simulink model "sistema"  (R2022a)
settings: Solver=ode1  StartTime=0.0  StopTime=tfinal  FixedStep=tstep  RelTol=1e-3
undefined symbols (not defined in the file or in its folder): ref_speed, wp_index_lim, wp_lat, wp_long, wp_time
libraries: robotmobilelib x1
settings Model: Creator=rodri  LastModifiedBy=rodri
settings DataIOCC: ExternalInput=[t2, u2]  SaveFormat=StructureWithTime  SignalLogging=off  DSMLogging=off  InspectSignalLogs=on  ReturnWorkspaceOutputs=off

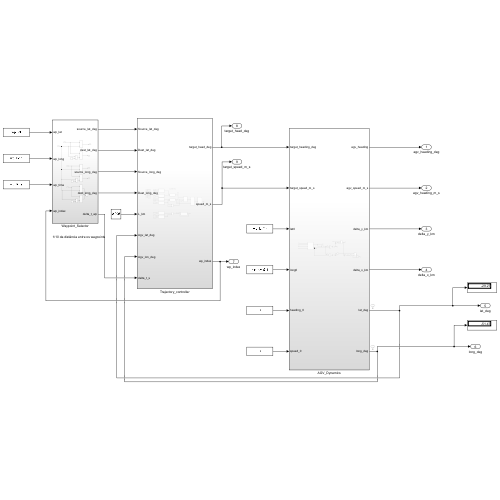
[thumbnail: Simulink's stored preview of the top-level diagram]
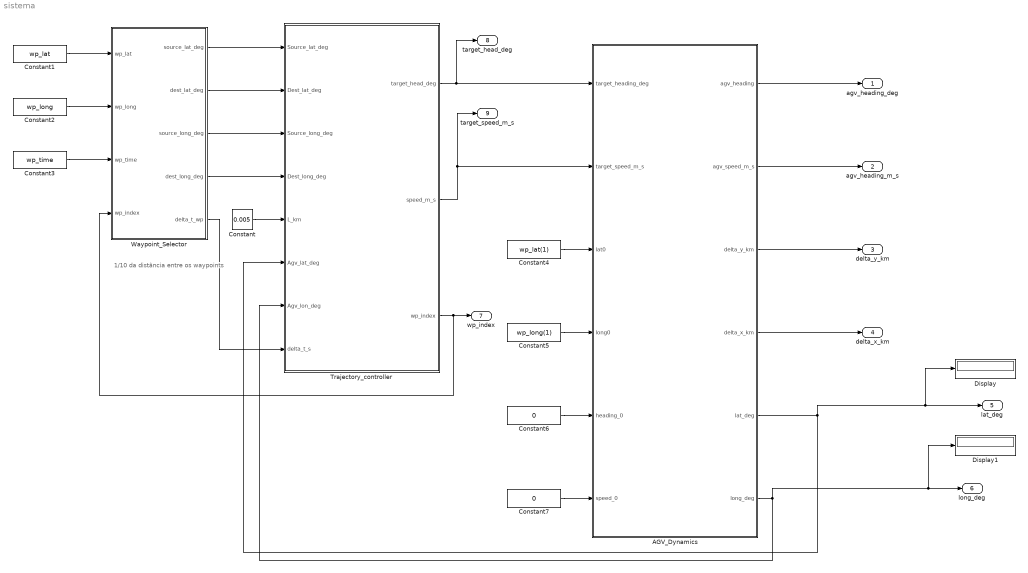
== system sistema ==
  note: 1/10 da distância entre os waypoints
  AGV_Dynamics : Subsystem
  Constant : Constant  Value=0.005
  Constant1 : Constant  Value=wp_lat
  Constant2 : Constant  Value=wp_long
  Constant3 : Constant  Value=wp_time
  Constant4 : Constant  Value=wp_lat(1)
  Constant5 : Constant  Value=wp_long(1)
  Constant6 : Constant  Value=0
  Constant7 : Constant  Value=0
  Display : Display
  Display1 : Display
  Trajectory_controller : Subsystem
  Waypoint_Selector : Subsystem
  agv_heading_deg : Outport
  agv_heading_m_s : Outport  Port=2
  delta_y_km : Outport  Port=3
  delta_x_km : Outport  Port=4
  lat_deg : Outport  Port=5
  long_deg : Outport  Port=6
  wp_index : Outport  Port=7
  target_head_deg : Outport  Port=8
  target_speed_m_s : Outport  Port=9
  wires:
  Waypoint_Selector/1(source_lat_deg) -> Trajectory_controller/1(Source_lat_deg)
  Waypoint_Selector/2(dest_lat_deg) -> Trajectory_controller/2(Dest_lat_deg)
  Waypoint_Selector/3(source_long_deg) -> Trajectory_controller/3(Source_long_deg)
  Waypoint_Selector/4(dest_long_deg) -> Trajectory_controller/4(Dest_long_deg)
  Constant/1 -> Trajectory_controller/5(L_km)
  Constant1/1 -> Waypoint_Selector/1(wp_lat)
  Constant2/1 -> Waypoint_Selector/2(wp_long)
  Constant3/1 -> Waypoint_Selector/3(wp_time)
  Waypoint_Selector/5(delta_t_wp) -> Trajectory_controller/8(delta_t_s)
  Trajectory_controller/3(wp_index) -> Waypoint_Selector/4(wp_index), wp_index/1
  Trajectory_controller/1(target_head_deg) -> target_head_deg/1, AGV_Dynamics/1(target_heading_deg)
  Trajectory_controller/2(speed_m_s) -> target_speed_m_s/1, AGV_Dynamics/2(target_speed_m_s)
  AGV_Dynamics/5(lat_deg) -> Display/1, lat_deg/1, Trajectory_controller/6(Agv_lat_deg)
  AGV_Dynamics/6(long_deg) -> Display1/1, long_deg/1, Trajectory_controller/7(Agv_lon_deg)
  AGV_Dynamics/1(agv_heading) -> agv_heading_deg/1
  AGV_Dynamics/2(agv_speed_m_s) -> agv_heading_m_s/1
  AGV_Dynamics/3(delta_y_km) -> delta_y_km/1
  AGV_Dynamics/4(delta_x_km) -> delta_x_km/1
  Constant4/1 -> AGV_Dynamics/3(lat0)
  Constant5/1 -> AGV_Dynamics/4(long0)
  Constant6/1 -> AGV_Dynamics/5(heading_0)
  Constant7/1 -> AGV_Dynamics/6(speed_0)

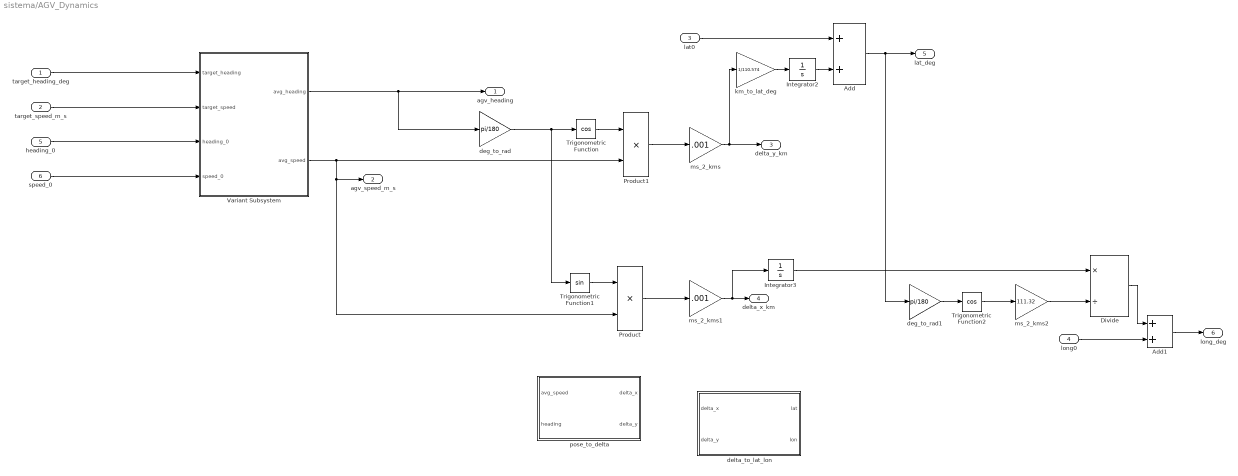
== system sistema/AGV_Dynamics ==
  target_heading_deg : Inport
  target_speed_m_s : Inport  Port=2
  lat0 : Inport  Port=3
  long0 : Inport  Port=4
  heading_0 : Inport  Port=5
  speed_0 : Inport  Port=6
  Add : Sum
  Add1 : Sum
  Divide : Product  Inputs=*/
  Integrator2 : Integrator
  Integrator3 : Integrator
  Product : Product
  Product1 : Product
  Trigonometric Function : Trigonometry  Operator=cos
  Trigonometric Function1 : Trigonometry
  Trigonometric Function2 : Trigonometry  Operator=cos
  Variant Subsystem : Subsystem  Variant=on
  deg_to_rad : Gain  Gain=pi/180
  deg_to_rad1 : Gain  Gain=pi/180
  delta_to_lat_lon : MATLAB Function  TreatAsAtomicUnit=on
  km_to_lat_deg : Gain  Gain=1/110.574
  ms_2_kms : Gain  Gain=.001
  ms_2_kms1 : Gain  Gain=.001
  ms_2_kms2 : Gain  Gain=111.32
  pose_to_delta : MATLAB Function  TreatAsAtomicUnit=on
  agv_heading : Outport
  agv_speed_m_s : Outport  Port=2
  delta_y_km : Outport  Port=3
  delta_x_km : Outport  Port=4
  lat_deg : Outport  Port=5
  long_deg : Outport  Port=6
  wires:
  deg_to_rad/1 -> Trigonometric Function1/1, Trigonometric Function/1
  Trigonometric Function1/1 -> Product/1
  Product/1 -> ms_2_kms1/1
  Trigonometric Function/1 -> Product1/1
  Product1/1 -> ms_2_kms/1
  ms_2_kms/1 -> delta_y_km/1, km_to_lat_deg/1
  ms_2_kms1/1 -> Integrator3/1, delta_x_km/1
  lat0/1 -> Add/1
  km_to_lat_deg/1 -> Integrator2/1
  Add/1 -> deg_to_rad1/1, lat_deg/1
  deg_to_rad1/1 -> Trigonometric Function2/1
  Trigonometric Function2/1 -> ms_2_kms2/1
  long0/1 -> Add1/2
  Divide/1 -> Add1/1
  ms_2_kms2/1 -> Divide/2
  Add1/1 -> long_deg/1
  Integrator3/1 -> Divide/1
  Integrator2/1 -> Add/2
  Variant Subsystem/1(avg_heading) -> deg_to_rad/1, agv_heading/1
  Variant Subsystem/2(avg_speed) -> Product/2, agv_speed_m_s/1, Product1/2
  target_heading_deg/1 -> Variant Subsystem/1(target_heading)
  target_speed_m_s/1 -> Variant Subsystem/2(target_speed)
  heading_0/1 -> Variant Subsystem/3(heading_0)
  speed_0/1 -> Variant Subsystem/4(speed_0)

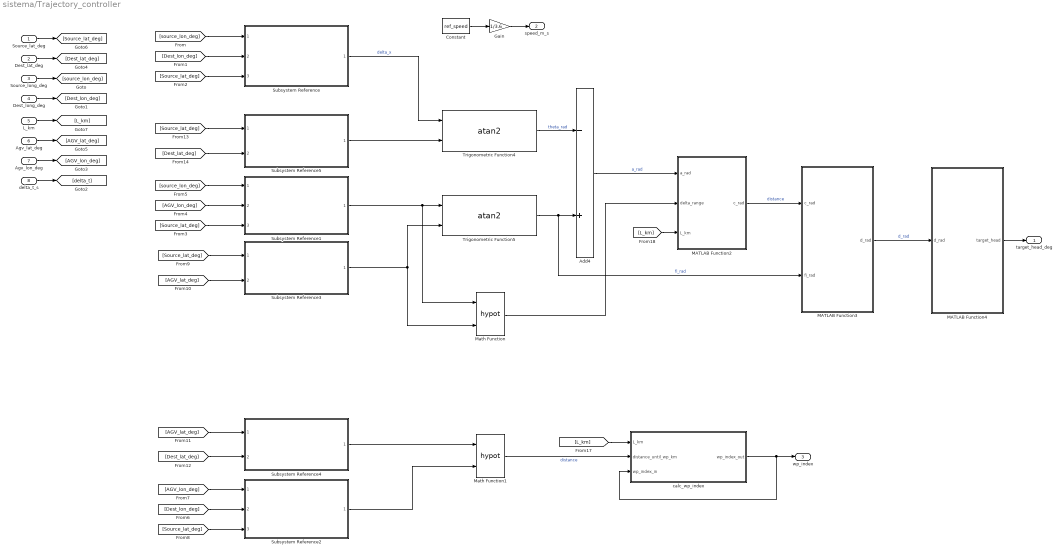
== system sistema/Trajectory_controller ==
  Source_lat_deg : Inport
  Dest_lat_deg : Inport  Port=2
  Source_long_deg : Inport  Port=3
  Dest_long_deg : Inport  Port=4
  L_km : Inport  Port=5
  Agv_lat_deg : Inport  Port=6
  Agv_lon_deg : Inport  Port=7
  delta_t_s : Inport  Port=8
  Add4 : Sum  Inputs=-+
  Constant : Constant  Value=ref_speed
  Gain : Gain  Gain=1/3.6
  MATLAB Function2 : MATLAB Function  TreatAsAtomicUnit=on
  MATLAB Function3 : MATLAB Function  TreatAsAtomicUnit=on
  MATLAB Function4 : MATLAB Function  TreatAsAtomicUnit=on
  Math Function : Math  Operator=hypot
  Math Function1 : Math  Operator=hypot
  Subsystem Reference : Subsystem  ReferencedSubsystem=long_deg_to_km
  Subsystem Reference1 : Subsystem  ReferencedSubsystem=long_deg_to_km
  Subsystem Reference2 : Subsystem  ReferencedSubsystem=long_deg_to_km
  Subsystem Reference3 : Subsystem  ReferencedSubsystem=lat_deg_to_km
  Subsystem Reference4 : Subsystem  ReferencedSubsystem=lat_deg_to_km
  Subsystem Reference5 : Subsystem  ReferencedSubsystem=lat_deg_to_km
  Trigonometric Function4 : Trigonometry  Operator=atan2
  Trigonometric Function5 : Trigonometry  Operator=atan2
  calc_wp_index : Subsystem
  target_head_deg : Outport
  speed_m_s : Outport  Port=2  Unit=m/s
  wp_index : Outport  Port=3
  wires:
  MATLAB Function4/1(target_head) -> target_head_deg/1
  Math Function1/1 -> calc_wp_index/2(distance_until_wp_km)  "distance"
  calc_wp_index/1(wp_index_out) -> calc_wp_index/3(wp_index_in), wp_index/1
  [source_lon_deg] -> Subsystem Reference/1
  [Dest_lon_deg] -> Subsystem Reference/2
  [Source_lat_deg] -> Subsystem Reference/3
  [Source_lat_deg] -> Subsystem Reference1/3
  [AGV_lon_deg] -> Subsystem Reference1/2
  [source_lon_deg] -> Subsystem Reference1/1
  [Dest_lon_deg] -> Subsystem Reference2/2
  [AGV_lon_deg] -> Subsystem Reference2/1
  [Source_lat_deg] -> Subsystem Reference2/3
  [Source_lat_deg] -> Subsystem Reference3/1
  [AGV_lat_deg] -> Subsystem Reference3/2
  [Dest_lat_deg] -> Subsystem Reference4/2
  [AGV_lat_deg] -> Subsystem Reference4/1
  Gain/1 -> speed_m_s/1
  [Source_lat_deg] -> Subsystem Reference5/1
  [Dest_lat_deg] -> Subsystem Reference5/2
  Trigonometric Function4/1 -> Add4/1  "theta_rad"
  Trigonometric Function5/1 -> MATLAB Function3/2(fi_rad), Add4/2  "fi_rad"
  Source_long_deg/1 -> [source_lon_deg]
  Dest_long_deg/1 -> [Dest_lon_deg]
  Source_lat_deg/1 -> [Source_lat_deg]
  Dest_lat_deg/1 -> [Dest_lat_deg]
  Agv_lat_deg/1 -> [AGV_lat_deg]
  Agv_lon_deg/1 -> [AGV_lon_deg]
  delta_t_s/1 -> [delta_t]
  L_km/1 -> [L_km]
  Subsystem Reference/1 -> Trigonometric Function4/1  "delta_x"
  Subsystem Reference5/1 -> Trigonometric Function4/2
  Subsystem Reference1/1 -> Math Function/1, Trigonometric Function5/1
  Subsystem Reference3/1 -> Math Function/2, Trigonometric Function5/2
  Subsystem Reference4/1 -> Math Function1/1
  Subsystem Reference2/1 -> Math Function1/2
  [L_km] -> calc_wp_index/1(L_km)
  Add4/1 -> MATLAB Function2/1(a_rad)  "a_rad"
  MATLAB Function2/1(c_rad) -> MATLAB Function3/1(c_rad)  "distance"
  Math Function/1 -> MATLAB Function2/2(delta_range)
  [L_km] -> MATLAB Function2/3(L_km)
  MATLAB Function3/1(d_rad) -> MATLAB Function4/1(d_rad)  "d_rad"
  Constant/1 -> Gain/1

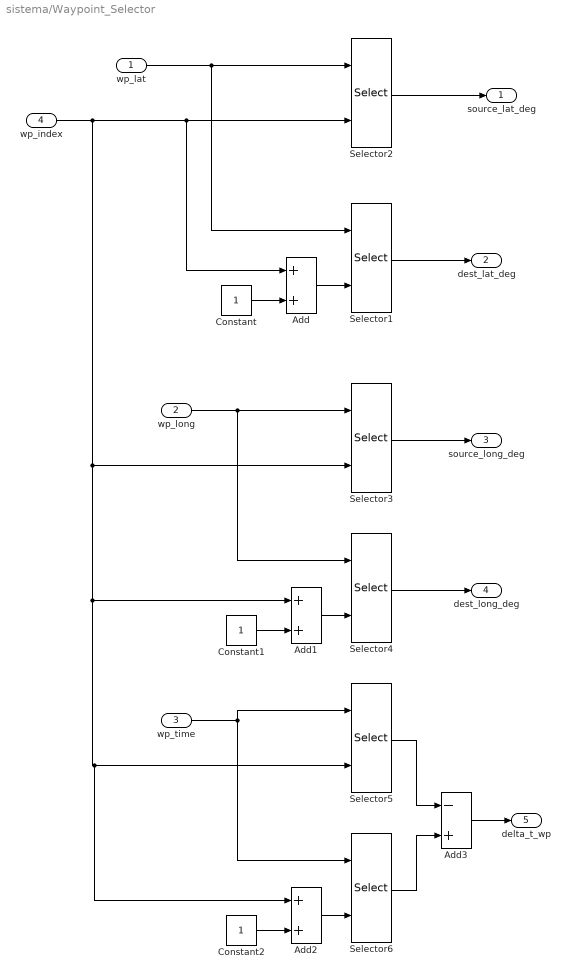
== system sistema/Waypoint_Selector ==
  wp_lat : Inport
  wp_long : Inport  Port=2
  wp_time : Inport  Port=3
  wp_index : Inport  Port=4
  Add : Sum
  Add1 : Sum
  Add2 : Sum
  Add3 : Sum  Inputs=-+
  Constant : Constant
  Constant1 : Constant
  Constant2 : Constant
  Selector{1..6} (6 alike) : Selector  InputPortWidth=num_of_wps  IndexOptions=Index vector (port)  Indices=[1 3]  OutputSizes=1
  source_lat_deg : Outport
  dest_lat_deg : Outport  Port=2
  source_long_deg : Outport  Port=3
  dest_long_deg : Outport  Port=4
  delta_t_wp : Outport  Port=5
  wires:
  Selector2/1 -> source_lat_deg/1
  Selector1/1 -> dest_lat_deg/1
  wp_lat/1 -> Selector2/1, Selector1/1
  Add/1 -> Selector1/2
  Constant/1 -> Add/2
  Selector3/1 -> source_long_deg/1
  Selector4/1 -> dest_long_deg/1
  wp_long/1 -> Selector4/1, Selector3/1
  Constant1/1 -> Add1/2
  Add1/1 -> Selector4/2
  Add2/1 -> Selector6/2
  Constant2/1 -> Add2/2
  wp_time/1 -> Selector5/1, Selector6/1
  wp_index/1 -> Add2/1, Selector5/2, Add1/1, Selector3/2, Selector2/2, Add/1
  Selector5/1 -> Add3/1
  Selector6/1 -> Add3/2
  Add3/1 -> delta_t_wp/1

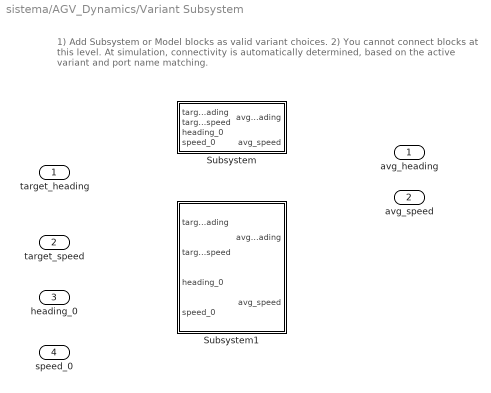
== system sistema/AGV_Dynamics/Variant Subsystem ==
  note: 1) Add Subsystem or Model blocks as valid variant choices.
      | 2) You cannot connect blocks at this level. At simulation, connectivity is automatically
      | determined, based on the active variant and port name matching.
  target_heading : Inport  Unit=deg
  target_speed : Inport  Port=2  Unit=m/s
  heading_0 : Inport  Port=3  Unit=m/s
  speed_0 : Inport  Port=4  Unit=m/s
  Subsystem : Subsystem  VariantControl=DYNMODE == 1
  Subsystem1 : Subsystem  VariantControl=DYNMODE == 2
  avg_heading : Outport
  avg_speed : Outport  Port=2

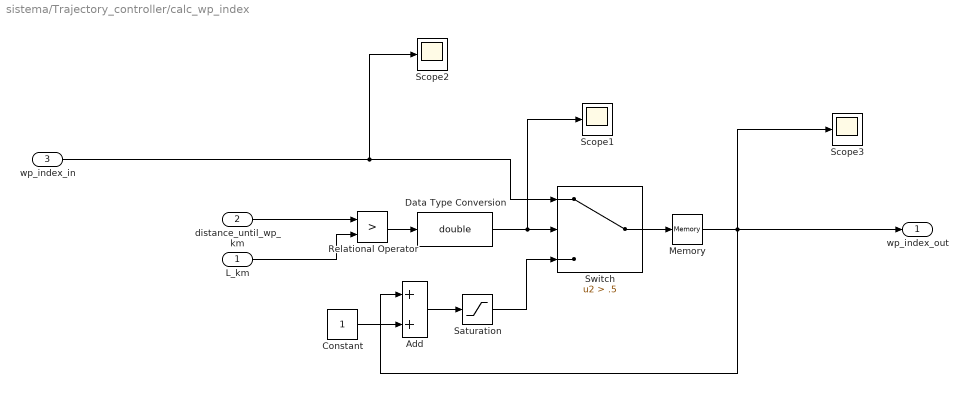
== system sistema/Trajectory_controller/calc_wp_index ==
  L_km : Inport
  distance_until_wp_km : Inport  Port=2
  wp_index_in : Inport  Port=3
  Add : Sum
  Constant : Constant
  Data Type Conversion : DataTypeConversion  OutDataTypeStr=double  SaturateOnIntegerOverflow=off  RndMeth=Floor
  Memory : Memory  InitialCondition=1
  Relational Operator : RelationalOperator  Operator=>  OutDataTypeStr=boolean  RndMeth=Simplest  InputSameDT=off
  Saturation : Saturate  UpperLimit=wp_index_lim  LowerLimit=1
  Scope1 : Scope
  Scope2 : Scope
  Scope3 : Scope
  Switch : Switch  Criteria=u2 > Threshold  Threshold=.5  SaturateOnIntegerOverflow=off  InputSameDT=off
  wp_index_out : Outport
  wires:
  distance_until_wp_km/1 -> Relational Operator/1
  L_km/1 -> Relational Operator/2
  Relational Operator/1 -> Data Type Conversion/1
  Data Type Conversion/1 -> Scope1/1, Switch/2
  Switch/1 -> Memory/1
  Memory/1 -> Add/1, Scope3/1, wp_index_out/1
  wp_index_in/1 -> Scope2/1, Switch/1
  Add/1 -> Saturation/1
  Constant/1 -> Add/2
  Saturation/1 -> Switch/3

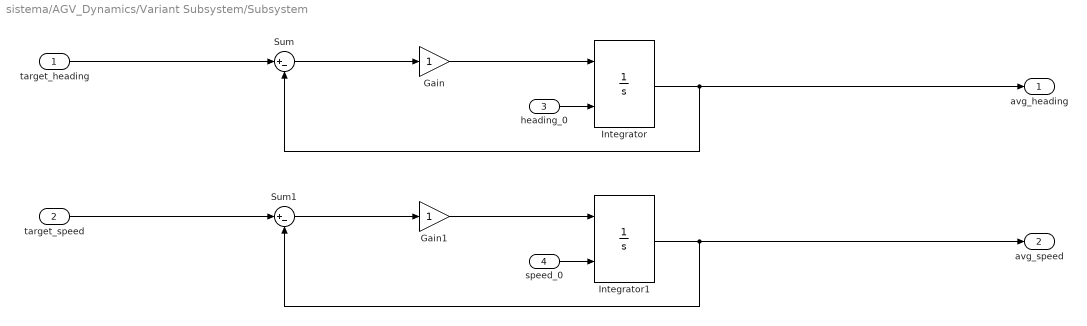
== system sistema/AGV_Dynamics/Variant Subsystem/Subsystem ==
  target_heading : Inport
  target_speed : Inport  Port=2
  heading_0 : Inport  Port=3
  speed_0 : Inport  Port=4
  Gain : Gain
  Gain1 : Gain
  Integrator : Integrator  InitialConditionSource=external
  Integrator1 : Integrator  InitialConditionSource=external
  Sum : Sum  Inputs=|+-
  Sum1 : Sum  Inputs=|+-
  avg_heading : Outport
  avg_speed : Outport  Port=2
  wires:
  target_speed/1 -> Sum1/1
  heading_0/1 -> Integrator/2
  Sum/1 -> Gain/1
  target_heading/1 -> Sum/1
  Integrator1/1 -> Sum1/2, avg_speed/1
  Gain1/1 -> Integrator1/1
  Sum1/1 -> Gain1/1
  Integrator/1 -> avg_heading/1, Sum/2
  Gain/1 -> Integrator/1
  speed_0/1 -> Integrator1/2

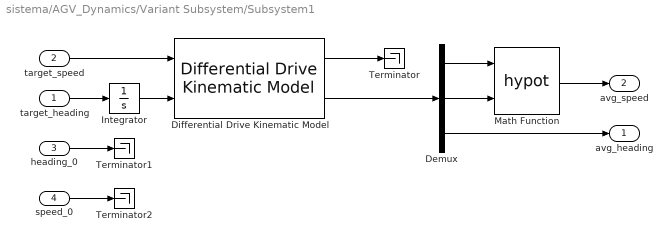
== system sistema/AGV_Dynamics/Variant Subsystem/Subsystem1 ==
  target_heading : Inport
  target_speed : Inport  Port=2
  heading_0 : Inport  Port=3
  speed_0 : Inport  Port=4
  Demux : Demux  Outputs=3
  Differential Drive Kinematic Model : robotmobilelib/Differential Drive Kinematic Model  VehicleInputs=Vehicle Speed & Heading Angular Velocity  WheelRadius=0.05  WheelSpeedRange=[-18, 18]  TrackWidth=0.8  InitialState=[0; 0; 0]  SimulateUsing=Interpreted execution
      settings: SourceProductBaseCode=RO
  Integrator : Integrator
  Math Function : Math  Operator=hypot
  Terminator : Terminator
  Terminator1 : Terminator
  Terminator2 : Terminator
  avg_heading : Outport
  avg_speed : Outport  Port=2
  wires:
  Differential Drive Kinematic Model/1 -> Terminator/1
  Differential Drive Kinematic Model/2 -> Demux/1
  Demux/3 -> avg_heading/1
  Demux/2 -> Math Function/2
  Demux/1 -> Math Function/1
  Math Function/1 -> avg_speed/1
  heading_0/1 -> Terminator1/1
  speed_0/1 -> Terminator2/1
  target_heading/1 -> Integrator/1
  target_speed/1 -> Differential Drive Kinematic Model/1
  Integrator/1 -> Differential Drive Kinematic Model/2

== matlab function sistema/AGV_Dynamics/delta_to_lat_lon ==
  data: delta_x input; lat output; delta_y input; lon output
function [lat, lon] = fcn(delta_x, delta_y)
k = 1e-3;
delta_x = k*sin(deg2rad(heading))*avg_speed;
delta_y = k*cos(deg2rad(heading))*avg_speed;

== matlab function sistema/AGV_Dynamics/pose_to_delta ==
  data: avg_speed input; delta_x output; heading input; delta_y output
function [delta_x, delta_y] = fcn(avg_speed, heading)
k = 1e-3;
delta_x = k*sin(deg2rad(heading))*avg_speed;
delta_y = k*cos(deg2rad(heading))*avg_speed;

== matlab function sistema/Trajectory_controller/MATLAB Function2 ==
  data: a_rad input; c_rad output; delta_range input; L_km input
function c_rad = B2C_rad(a_rad, delta_range, L_km)

c_rad = pi - a_rad - asin(sin(a_rad)*delta_range/L_km);

end

== matlab function sistema/Trajectory_controller/MATLAB Function3 ==
  data: c_rad input; fi_rad input; d_rad output
function d_rad = D_rad(c_rad, fi_rad)

d_rad = pi - fi_rad - c_rad;
end

== matlab function sistema/Trajectory_controller/MATLAB Function4 ==
  data: d_rad input; target_head output
function target_head = Target_head(d_rad)

target_head = (2*pi - d_rad) * 180 / pi;
end
